simulink model "Part3"  (R2024a)
settings: Solver=VariableStepAuto  StartTime=0.0  StopTime=10  RelTol=1e-3
settings Model: Creator=kyleo  LastModifiedBy=kyleo

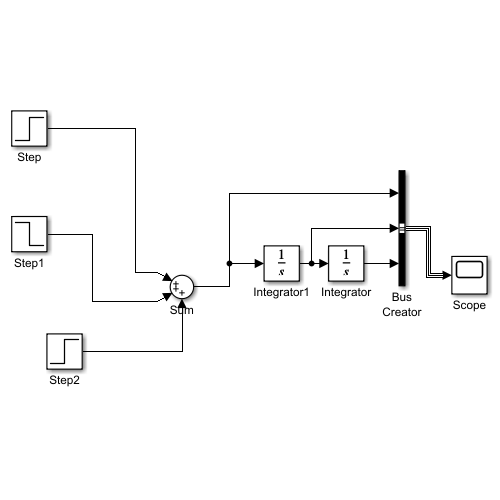
[thumbnail: Simulink's stored preview of the top-level diagram]
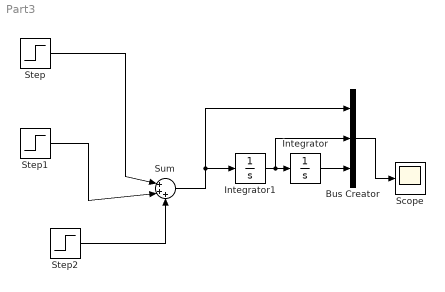
== system Part3 ==
  Bus Creator : BusCreator  Inputs=3
  Integrator : Integrator
  Integrator1 : Integrator
  Scope : Scope
  Step : Step  SampleTime=0
  Step1 : Step  Time=5  Before=1  After=-1  SampleTime=0
  Step2 : Step  Time=9  Before=-1  After=0  SampleTime=0
  Sum : Sum  Inputs=|+++
  wires:
  Step/1 -> Sum/1
  Step1/1 -> Sum/2
  Step2/1 -> Sum/3
  Integrator/1 -> Bus Creator/3
  Integrator1/1 -> Bus Creator/2, Integrator/1
  Sum/1 -> Bus Creator/1, Integrator1/1
  Bus Creator/1 -> Scope/1
